simulink model "ctsdm_3stage_NRZ_DAC"  (R2021a)
settings: Solver=VariableStepAuto  StartTime=0.0  StopTime=time  RelTol=1e-3
undefined symbols (not defined in the file or in its folder): c1, c2, c3, fin, fs, k1, k2, k3, n, osr, Td, Ts
libraries: SDtoolbox x1
settings Model: Creator=weihaoyu  LastModifiedBy=weihaoyu

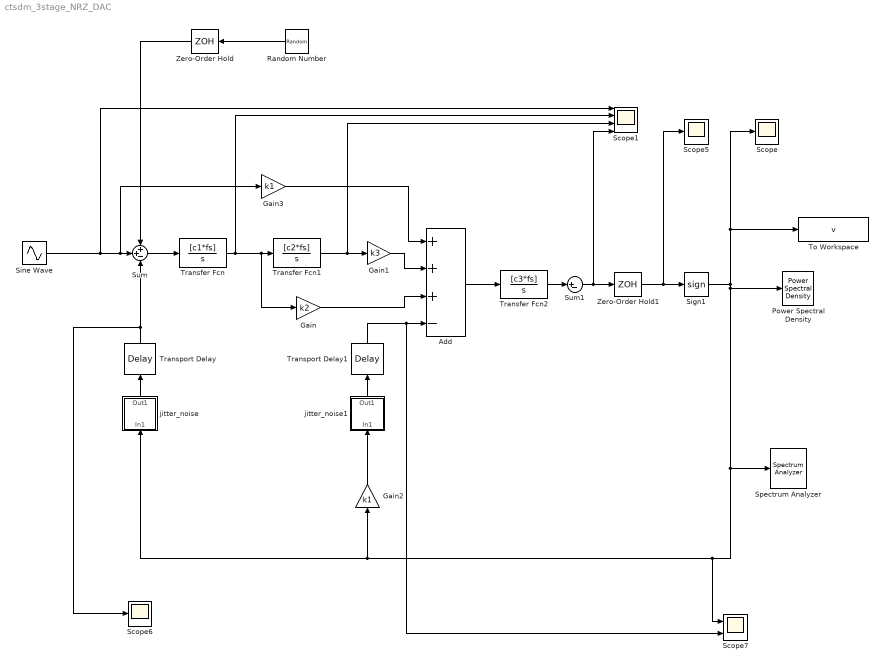
== system ctsdm_3stage_NRZ_DAC ==
  Add : Sum  Inputs=+++-
  Gain : Gain  Gain=k2
  Gain1 : Gain  Gain=k3
  Gain2 : Gain  Gain=k1
  Gain3 : Gain  Gain=k1
  Power Spectral Density : SDtoolbox/Power Spectral Density  SN=2  Fs=fs  fBL=0  fBH=fs/(2*osr)  Fin=fin  N=n  Ntransient=0  VW=off  savename=savemat  Scale_type=logarithmic
  Random Number : RandomNumber  Variance=6.91e-6^2  SampleTime=Ts
  Scope : Scope
  Scope1 : Scope  NumInputPorts=4
  Scope5 : Scope
  Scope6 : Scope
  Scope7 : Scope  NumInputPorts=2
  Sign1 : Signum
  Sine Wave : Sin  Amplitude=0.8  Frequency=fin*2*pi  SampleTime=0
  Spectrum Analyzer : SpectrumAnalyzer
  Sum : Sum  Inputs=++-
  Sum1 : Sum  Inputs=|+-
  To Workspace : ToWorkspace  VariableName=v  SampleTime=1/fs
  Transfer Fcn : TransferFcn  Numerator=[c1*fs]  Denominator=[1 0]
  Transfer Fcn1 : TransferFcn  Numerator=[c2*fs]  Denominator=[1 0]
  Transfer Fcn2 : TransferFcn  Numerator=[c3*fs]  Denominator=[1 0]
  Transport Delay : TransportDelay  DelayTime=Td
  Transport Delay1 : TransportDelay  DelayTime=Td
  Zero-Order Hold : ZeroOrderHold  SampleTime=-1
  Zero-Order Hold1 : ZeroOrderHold  SampleTime=1/fs
  jitter_noise : Subsystem
  jitter_noise1 : Subsystem
  wires:
  Transfer Fcn/1 -> Scope1/2, Gain/1, Transfer Fcn1/1
  Transfer Fcn1/1 -> Scope1/3, Gain1/1
  Gain1/1 -> Add/2
  Gain/1 -> Add/3
  Add/1 -> Transfer Fcn2/1
  Gain2/1 -> jitter_noise1/1(In1)
  Sine Wave/1 -> Scope1/1, Gain3/1, Sum/2
  Sum/1 -> Transfer Fcn/1
  Gain3/1 -> Add/1
  Zero-Order Hold1/1 -> Sign1/1, Scope5/1
  Transfer Fcn2/1 -> Sum1/1
  Sum1/1 -> Scope1/4, Zero-Order Hold1/1
  Random Number/1 -> Zero-Order Hold/1
  Zero-Order Hold/1 -> Sum/1
  Sign1/1 -> Power Spectral Density/1, Scope7/1, jitter_noise/1(In1), Gain2/1, Spectrum Analyzer/1, To Workspace/1, Scope/1
  Transport Delay/1 -> Scope6/1, Sum/3
  Transport Delay1/1 -> Add/4, Scope7/2
  jitter_noise/1(Out1) -> Transport Delay/1
  jitter_noise1/1(Out1) -> Transport Delay1/1

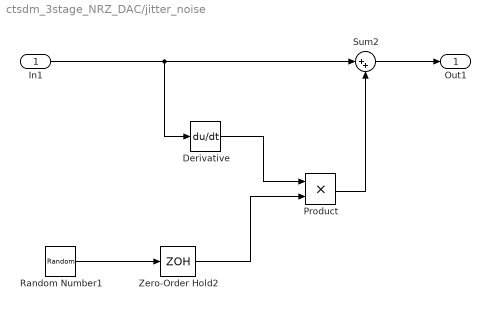
== system ctsdm_3stage_NRZ_DAC/jitter_noise ==
  In1 : Inport
  Derivative : Derivative
  Product : Product
  Random Number1 : RandomNumber  Variance=(4e-4*Ts)^2  SampleTime=Ts
  Sum2 : Sum  Inputs=|++
  Zero-Order Hold2 : ZeroOrderHold  SampleTime=-1
  Out1 : Outport
  wires:
  Sum2/1 -> Out1/1
  Derivative/1 -> Product/1
  In1/1 -> Derivative/1, Sum2/1
  Random Number1/1 -> Zero-Order Hold2/1
  Zero-Order Hold2/1 -> Product/2
  Product/1 -> Sum2/2

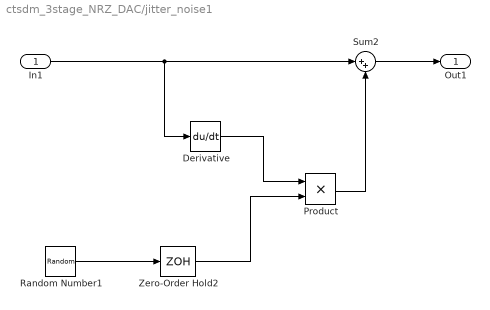
== system ctsdm_3stage_NRZ_DAC/jitter_noise1 ==
  In1 : Inport
  Derivative : Derivative
  Product : Product
  Random Number1 : RandomNumber  Variance=(4e-4*Ts)^2  SampleTime=Ts
  Sum2 : Sum  Inputs=|++
  Zero-Order Hold2 : ZeroOrderHold  SampleTime=-1
  Out1 : Outport
  wires:
  Product/1 -> Sum2/2
  Zero-Order Hold2/1 -> Product/2
  Random Number1/1 -> Zero-Order Hold2/1
  In1/1 -> Sum2/1, Derivative/1
  Derivative/1 -> Product/1
  Sum2/1 -> Out1/1
